simulink model "slexPRFSelectionSEExample"  (R2018b)
settings: Solver=VariableStepDiscrete  StartTime=0.0  StopTime=0.2  RelTol=1e-3  EnableMultiTasking=on
PreLoadFcn:
  | load radarTask
  | helperslexPRFSelectionParam
undefined symbols (not defined in the file or in its folder): m, paramPRFSel
libraries: phasedenvlib x4, phaseddetectlib x3, phasedtxrxlib x2, phasedwavlib x1
CloseFcn:
  | clear paramPRFSel
  | clear radarTask
settings Model: Creator=The MathWorks, Inc.  LastModifiedBy=The MathWorks, Inc.
settings DataIOCC: SaveFormat=Array
settings OptimizationCC: LifeSpan=inf
settings DebuggingCC: SFUnexpectedBacktrackingDiag=warning  SFNoUnconditionalDefaultTransitionDiag=warning  SFExecutionAtInitializationDiag=none
settings ModelReferenceCC: PropagateSignalLabelsOutOfModel=off
settings SFSimCC: SimUseLocalCustomCode=off
settings RTWCC: RTWUseLocalCustomCode=off
settings CodeAppCC: StateflowObjectComments=on
settings GRTTargetCC: TargetLangStandard=C89/C90 (ANSI)  GeneratePreprocessorConditionals=Disable all
settings ConfigComp: CovMetricSettings=dw  CovHtmlReporting=on  CovSaveCumulativeToWorkspaceVar=on  CovSaveSingleToWorkspaceVar=on  CovShowResultsExplorer=off  CovExternalEMLEnable=off

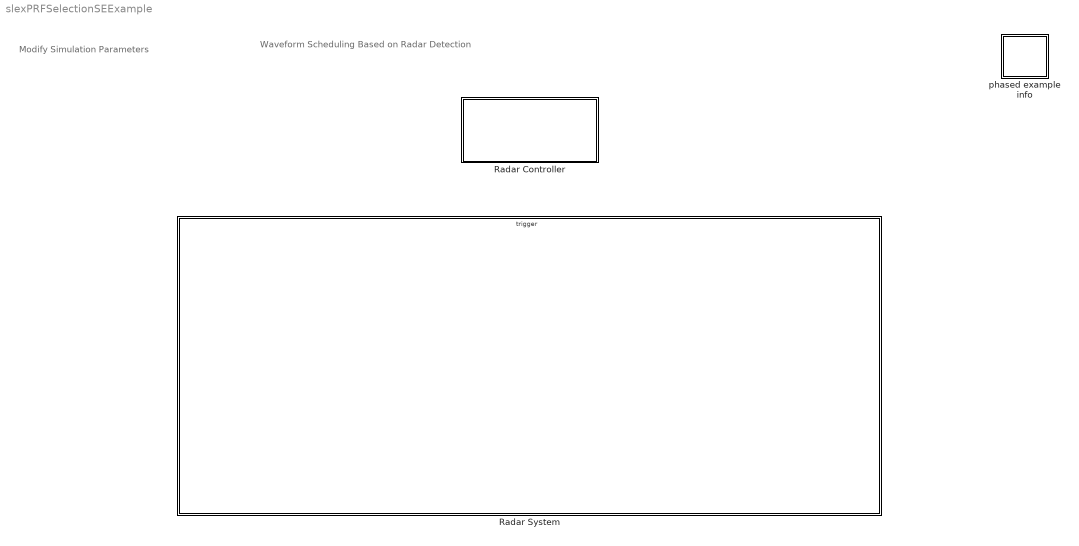
== system slexPRFSelectionSEExample ==
  note: Waveform Scheduling Based on Radar Detection
  note: Modify Simulation Parameters
  Radar Controller : Subsystem
  Radar System : Subsystem  TreatAsAtomicUnit=on
  phased example info : Subsystem
      settings: OpenFcn=|
      | modelname = 'slexPRFSelectionSEExample';
      | helpview(fullfile(matlabroot,'help','phased','helptargets.map'),sprintf('%sExample',modelname));
      | clear modelname;
      mask Display: disp('Info')

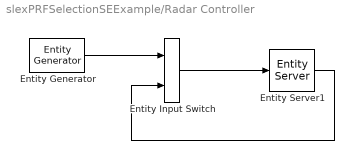
== system slexPRFSelectionSEExample/Radar Controller ==
  Entity Input Switch : EntityInputSwitch  InputPortMessageModes=m,m  OutputPortMessageModes=m
  Entity Generator : EntityGenerator  OutputPortMessageModes=m  Period=inf  GenerateAction=|  EntityType=Bus object  EntityTypeName=radarTask
      | entity.idx = 1;
      | entity.dt = 0;
  Entity Server1 : EntityServer  InputPortMessageModes=m  OutputPortMessageModes=m  Capacity=2  ServiceTimeSource=Attribute  ServiceTimeAttributeName=dt  EntryAction=[entity.dt, entity.r] = f(entity.idx);  ServiceCompleteAction=|
      | if entity.r < 2000
      |     entity.idx = 2;
      | else
      |     entity.idx = 1;
      | end
  wires:
  Entity Generator/1 -> Entity Input Switch/1
  Entity Input Switch/1 -> Entity Server1/1
  Entity Server1/1 -> Entity Input Switch/2

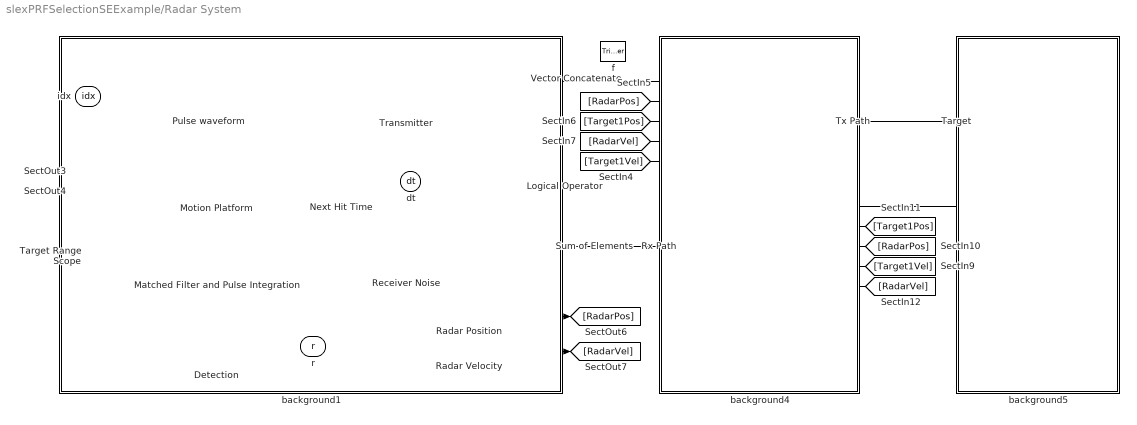
== system slexPRFSelectionSEExample/Radar System ==
  f : TriggerPort  TriggerType=function-call  IsSimulinkFunction=on  FunctionName=f  VariantControl=Variant
  Detection : MATLAB Function  TreatAsAtomicUnit=on  mask{dr=paramPRFSel.metersPerSample}
      mask prompts: dr "Range Increment (m)"
  Logical Operator : Logic  Operator=NOT  AllPortsSameDT=off  OutDataTypeStr=boolean
  Matched Filter and Pulse Integration : Subsystem
      mask Display: disp('Signal Processing')
  Motion Platform : phasedenvlib/Motion Platform  MotionModel=Velocity  InitialPosition=paramPRFSel.target1Pos  InitialVelocity=[ 0; 0; 0 ]  VelocitySource=Property  Velocity=paramPRFSel.target1Vel  AccelerationSource=Property  Acceleration=[0;0;0]  CustomTrajectory=[ 0, 0, 0, 0, 0, 0, 0; 1, 0, 0, 0, 0, 0, 0 ]  ScanMode=None  InitialScanAngle=0  AzimuthSpan=[ -60, 60 ]  AzimuthScanRate=10  InitialOrientationAxes=eye( 3 )  OrientationAxesOutputPort=off  ElapsedTimeSource=Derive from reference input port  SampleRateFromInputCheckbox=off  SampleRate=paramPRFSel.fs  SimulateUsing=Interpreted execution
      settings: SourceProductName=Phased Array System Toolbox  SourceProductBaseCode=AR
  Next Hit Time : MATLAB Function  TreatAsAtomicUnit=on  mask{fs=paramPRFSel.fs}
      mask prompts: fs "Sample rate"
  Pulse waveform : phasedwavlib/Rectangular Waveform  SampleRate=paramPRFSel.fs  DurationSpecification=Pulse width  PulseWidth=1/paramPRFSel.pulseBw  DutyCycle=0.5  PRF=paramPRFSel.prf  PRFSelectionInputPort=on  SimulationTimeSource=Inherit from Simulink engine  OutputFormat=Pulses  NumSamples=100  NumPulses=1  PRFOutputPort=off  SimulateUsing=Interpreted execution
      settings: SourceProductName=Phased Array System Toolbox  SourceProductBaseCode=AR
  Radar Position : Constant  Value=[ 0; 0; 0 ]  SampleTime=-1
  Radar Velocity : Constant  Value=[ 0; 0; 0 ]  SampleTime=-1
  Receiver Noise : phasedtxrxlib/Receiver Preamp  Gain=20  LossFactor=0  NoiseMethod=Noise temperature  NoiseFigure=0  ReferenceTemperature=290  SampleRateFromInputCheckbox=off  SampleRate=paramPRFSel.fs  NoisePower=0  EnableInputPort=on  PhaseNoiseInputPort=off  SeedSource=Auto  Seed=0  SimulateUsing=Interpreted execution
      settings: SourceProductName=Phased Array System Toolbox  SourceProductBaseCode=AR
  Rx Path : phasedenvlib/Free Space  PropagationSpeed=paramPRFSel.propSpeed  OperatingFrequency=paramPRFSel.fc  TwoWayPropagation=off  SampleRateFromInputCheckbox=off  SampleRate=paramPRFSel.fs  MaximumDistanceSource=Property  MaximumDistance=10e3  MaximumNumInputSamplesSource=Auto  MaximumNumInputSamples=1000  SimulateUsing=Interpreted execution
      settings: SourceProductName=Phased Array System Toolbox  SourceProductBaseCode=AR
  Sum of Elements : Sum  Inputs=+  CollapseMode=Specified dimension  CollapseDim=2
  Target : phasedenvlib/Radar Target  EnablePolarization=off  Mode=Monostatic  MeanRCSSource=Property  ScatteringMatrixSource=Property  MeanRCS=paramPRFSel.target1Rcs  ScatteringMatrix=eye( 2 )  Model=Nonfluctuating  PropagationSpeed=paramPRFSel.propSpeed  OperatingFrequency=paramPRFSel.fc  SeedSource=Auto  Seed=0  SimulateUsing=Interpreted execution
      settings: SourceProductName=Phased Array System Toolbox  SourceProductBaseCode=AR
  Target Range Scope : ArrayPlot
  Transmitter : phasedtxrxlib/Transmitter  PeakPower=paramPRFSel.peakPower  Gain=paramPRFSel.txGain  LossFactor=0  InUseOutputPort=on  CoherentOnTransmit=on  PhaseNoiseOutputPort=off  SeedSource=Auto  Seed=0  SimulateUsing=Interpreted execution
      settings: SourceProductName=Phased Array System Toolbox  SourceProductBaseCode=AR
  Tx Path : phasedenvlib/Free Space  PropagationSpeed=paramPRFSel.propSpeed  OperatingFrequency=paramPRFSel.fc  TwoWayPropagation=off  SampleRateFromInputCheckbox=off  SampleRate=paramPRFSel.fs  MaximumDistanceSource=Property  MaximumDistance=10e3  MaximumNumInputSamplesSource=Auto  MaximumNumInputSamples=1000  SimulateUsing=Interpreted execution
      settings: SourceProductName=Phased Array System Toolbox  SourceProductBaseCode=AR
  Vector Concatenate : Concatenate  Mode=Multidimensional array  ConcatenateDimension=2
  background1 : Subsystem  Description=Jammer
      mask Display: disp('')
  background4 : Subsystem  Description=Jammer
      mask Display: disp('')
  background5 : Subsystem  Description=Jammer
      mask Display: disp('')
  idx : ArgIn  ArgumentName=idx
  dt : ArgOut  ArgumentName=dt
  r : ArgOut  Port=2  PortDimensions=[1 1]  ArgumentName=r
  wires:
  idx/1 -> Pulse waveform/1
  Next Hit Time/1(y) -> dt/1
  Detection/1(y) -> r/1
  Receiver Noise/1 -> Matched Filter and Pulse Integration/1(In1)
  Matched Filter and Pulse Integration/1(Out1) -> Detection/1(u), Target Range Scope/1
  Transmitter/2 -> Logical Operator/1
  Logical Operator/1 -> Receiver Noise/2
  [RadarVel] -> Tx Path/4
  [Target1Pos] -> Tx Path/3
  [Target1Vel] -> Tx Path/5
  [RadarPos] -> Tx Path/2
  [Target1Vel] -> Rx Path/4
  [Target1Pos] -> Rx Path/2
  [RadarPos] -> Rx Path/3
  [RadarVel] -> Rx Path/5
  Tx Path/1 -> Target/1
  Target/1 -> Rx Path/1
  Rx Path/1 -> Sum of Elements/1
  Radar Position/1 -> [RadarPos]
  Radar Velocity/1 -> [RadarVel]
  Pulse waveform/1 -> Motion Platform/1, Next Hit Time/1(u), Transmitter/1
  Motion Platform/1 -> [Target1Pos]
  Motion Platform/2 -> [Target1Vel]
  Transmitter/1 -> Vector Concatenate/2, Vector Concatenate/1
  Vector Concatenate/1 -> Tx Path/1
  Sum of Elements/1 -> Receiver Noise/1

== system slexPRFSelectionSEExample/phased example info ==

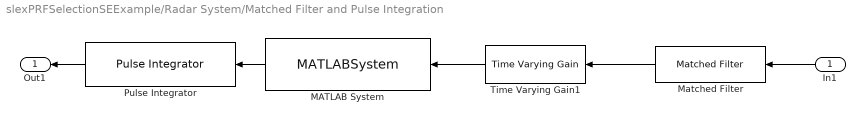
== system slexPRFSelectionSEExample/Radar System/Matched Filter and Pulse Integration ==
  In1 : Inport
  MATLAB System : MATLABSystem  System=phased.internal.SimulinkSignalPadder  SignalLengthOutputPort=off  SimulateUsing=Interpreted execution
      mask Type: phased.internal.SimulinkSignalPadder
      mask Display:
      | disp('Signal Padder');
      | port_label('input',1,'X');
      | port_label('output',1,'Xp');
  Matched Filter : phaseddetectlib/Matched Filter  CoefficientsSource=Property  Coefficients=paramPRFSel.matchingCoeff  SpectrumWindow=None  CustomSpectrumWindow=@hamming  SpectrumRange=[ 0, 1e5 ]  SampleRateFromInputCheckbox=on  SampleRate=1e6  SidelobeAttenuation=30  Beta=0.5  Nbar=4  GainOutputPort=off  MaximumNumInputSamplesSource=Auto  MaximumNumInputSamples=100  SimulateUsing=Interpreted execution
      settings: SourceProductName=Phased Array System Toolbox  SourceProductBaseCode=AR
  Pulse Integrator : phaseddetectlib/Pulse Integrator  CoherentFlag=Noncoherent  N=10  V=9
      settings: SourceProductName=Phased Array System Toolbox  SourceProductBaseCode=AR
  Time Varying Gain1 : phaseddetectlib/Time Varying Gain  RangeLossSource=Property  RangeLoss=paramPRFSel.rangeLoss  ReferenceLoss=paramPRFSel.referenceLoss  SimulateUsing=Interpreted execution
      settings: SourceProductName=Phased Array System Toolbox  SourceProductBaseCode=AR
  Out1 : Outport
  wires:
  In1/1 -> Matched Filter/1
  Time Varying Gain1/1 -> MATLAB System/1
  Matched Filter/1 -> Time Varying Gain1/1
  Pulse Integrator/1 -> Out1/1
  MATLAB System/1 -> Pulse Integrator/1

== system slexPRFSelectionSEExample/Radar System/background1 ==

== system slexPRFSelectionSEExample/Radar System/background4 ==

== system slexPRFSelectionSEExample/Radar System/background5 ==

== matlab function slexPRFSelectionSEExample/Radar System/Detection ==
  data: u input; y output; dr parameter
function y = fcn(u,dr)
%#codegen

%y = double(~rem(numel(u),2));
[~,idx] = max(u);
y = dr*(idx-1);

== matlab function slexPRFSelectionSEExample/Radar System/Next Hit Time ==
  data: u input; y output; fs parameter size=1
function y = fcn(u,fs)
%#codegen

y = numel(u)/fs;
